simulink model "CH22_5"  (R2021b)
settings: Solver=ode45  StartTime=0.0  StopTime=inf  RelTol=1e-3  EnableMultiTasking=on
values from neighbouring files (symbols this model uses):
  v_n = N0/(2*t_step)    [CH22_5C1.m]
libraries: simulink x2, commsink2 x2, commfilt2 x2, commrandsrc2 x2, commutil2 x2
settings Model: Creator=my2  LastModifiedBy=IT
settings SolverCC: AlgebraicLoopSolver=TrustRegion
settings DataIOCC: SaveFormat=Array  SignalLoggingSaveFormat=ModelDataLogs  ReturnWorkspaceOutputs=off
settings OptimizationCC: LifeSpan=inf
settings DebuggingCC: UnderspecifiedInitializationDetection=Classic  MergeDetectMultiDrivingBlocksExec=none  SolverPrmCheckMsg=warning  MultiTaskDSMMsg=warning  MultiTaskCondExecSysMsg=none  FcnCallInpInsideContextMsg=warning  SFUnexpectedBacktrackingDiag=warning  SFNoUnconditionalDefaultTransitionDiag=warning  SFExecutionAtInitializationDiag=none  SFMachineParentedDataDiag=warning  ArithmeticOperatorsInVariantConditions=warning
settings HardwareCC: ProdBitPerPointer=32  ProdBitPerSizeT=32  ProdBitPerPtrDiffT=32  ProdLargestAtomicFloat=None  ProdIntDivRoundTo=Undefined  ProdEndianess=Unspecified  ProdWordSize=32  ProdHWDeviceType=32-bit Generic
settings ModelReferenceCC: PropagateSignalLabelsOutOfModel=off
settings SFSimCC: SimUseLocalCustomCode=off  CustomCodeUndefinedFunction=UseInterfaceOnly
settings RTWCC: RTWUseLocalCustomCode=off
settings CodeAppCC: StateflowObjectComments=on
settings GRTTargetCC: TargetLangStandard=C89/C90 (ANSI)  CombineOutputUpdateFcns=off  GRTInterface=on
settings ConfigComp: CovMetricSettings=dw  CovSaveCumulativeToWorkspaceVar=on  CovSaveSingleToWorkspaceVar=on  CovExternalEMLEnable=off

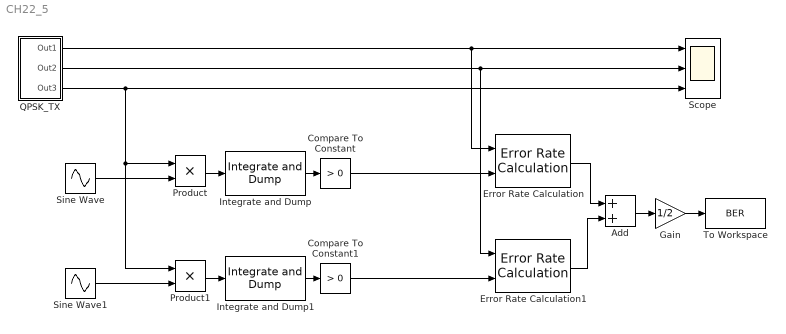
== system CH22_5 ==
  Add : Sum
  Compare To Constant : simulink/Logic and Bit Operations/Compare To Constant  relop=>  const=0  OutDataTypeStr=boolean
  Compare To Constant1 : simulink/Logic and Bit Operations/Compare To Constant  relop=>  const=0  OutDataTypeStr=boolean
  Error Rate Calculation : commsink2/Error Rate Calculation  N=1  st_delay=0  cp_mode=Entire frame  subframe=[]  PMode=Port  WsName=ErrorVec  RsMode2=off  stop=on  numErr=Nerrs  maxBits=inf
  Error Rate Calculation1 : commsink2/Error Rate Calculation  N=1  st_delay=0  cp_mode=Entire frame  subframe=[]  PMode=Port  WsName=ErrorVec  RsMode2=off  stop=on  numErr=Nerrs  maxBits=inf
  Gain : Gain  Gain=1/2
  Integrate and Dump : commfilt2/Integrate and Dump  obssamples=8  offsetsamples=0  nodump=off  roundingMode=Floor  overflowMode=off  outputDataTypeStr=Inherit: Same as accumulator  outputLastDataTypeStr=Inherit: Same as accumulator
  Integrate and Dump1 : commfilt2/Integrate and Dump  obssamples=8  offsetsamples=0  nodump=off  roundingMode=Floor  overflowMode=off  outputDataTypeStr=Inherit: Same as accumulator  outputLastDataTypeStr=Inherit: Same as accumulator
  Product : Product
  Product1 : Product
  QPSK_TX : Subsystem
  Scope : Scope  NumInputPorts=3
  Sine Wave : Sin  SampleTime=1/256
  Sine Wave1 : Sin  SampleTime=1/256
  To Workspace : ToWorkspace  VariableName=BER  SampleTime=-1
      settings: MaxDataPoints=1
  wires:
  Sine Wave/1 -> Product/2
  Product/1 -> Integrate and Dump/1
  QPSK_TX/3(Out3) -> Product/1, Product1/1, Scope/3
  Sine Wave1/1 -> Product1/2
  Product1/1 -> Integrate and Dump1/1
  Integrate and Dump/1 -> Compare To Constant/1
  Integrate and Dump1/1 -> Compare To Constant1/1
  QPSK_TX/1(Out1) -> Error Rate Calculation/1, Scope/1
  QPSK_TX/2(Out2) -> Error Rate Calculation1/1, Scope/2
  Error Rate Calculation/1 -> Add/1
  Error Rate Calculation1/1 -> Add/2
  Add/1 -> Gain/1
  Gain/1 -> To Workspace/1
  Compare To Constant/1 -> Error Rate Calculation/2
  Compare To Constant1/1 -> Error Rate Calculation1/2

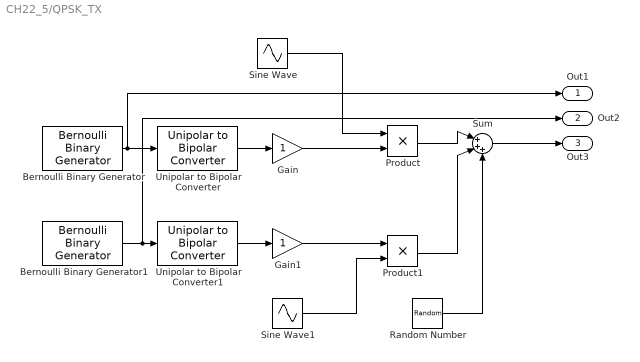
== system CH22_5/QPSK_TX ==
  Bernoulli Binary Generator : commrandsrc2/Bernoulli Binary Generator  P=0.5  seed=20301181  Ts=1  frameBased=off  sampPerFrame=1  orient=off  outDataType=boolean
      settings: SourceProductBaseCode=CM
  Bernoulli Binary Generator1 : commrandsrc2/Bernoulli Binary Generator  P=0.5  seed=7  Ts=1  frameBased=off  sampPerFrame=1  orient=off  outDataType=boolean
      settings: SourceProductBaseCode=CM
  Gain : Gain
  Gain1 : Gain
  Product : Product
  Product1 : Product
  Random Number : RandomNumber  Variance=v_n  Seed=41  SampleTime=1/256  VectorParams1D=off
  Sine Wave : Sin  SampleTime=1/256
  Sine Wave1 : Sin  SampleTime=1/256
  Sum : Sum  Inputs=|+++
  Unipolar to Bipolar Converter : commutil2/Unipolar to Bipolar Converter  M=2  polarity=Positive  dataType=Inherit via internal rule
  Unipolar to Bipolar Converter1 : commutil2/Unipolar to Bipolar Converter  M=2  polarity=Positive  dataType=Inherit via internal rule
  Out1 : Outport
  Out2 : Outport  Port=2
  Out3 : Outport  Port=3
  wires:
  Sum/1 -> Out3/1
  Unipolar to Bipolar Converter/1 -> Gain/1
  Sine Wave1/1 -> Product1/2
  Gain1/1 -> Product1/1
  Sine Wave/1 -> Product/1
  Bernoulli Binary Generator/1 -> Out1/1, Unipolar to Bipolar Converter/1
  Product/1 -> Sum/1
  Product1/1 -> Sum/2
  Unipolar to Bipolar Converter1/1 -> Gain1/1
  Bernoulli Binary Generator1/1 -> Out2/1, Unipolar to Bipolar Converter1/1
  Gain/1 -> Product/2
  Random Number/1 -> Sum/3
